simulink model "Plant_Simulation"  (R2024b)
settings: Solver=FixedStepAuto  StartTime=0.0  StopTime=10  FixedStep=5e-4  RelTol=1e-3
values from neighbouring files (symbols this model uses):
  ts = p.ctrl.ts_s    [discretization.m]
libraries: cstblocks x2
settings Model: Creator=HakvoortWBJ  LastModifiedBy=gicub
settings SolverCC: AlgebraicLoopSolver=TrustRegion
settings DataIOCC: ReturnWorkspaceOutputs=off
settings DebuggingCC: UnconnectedInputMsg=warning  UnconnectedOutputMsg=warning  UnconnectedLineMsg=warning  ArithmeticOperatorsInVariantConditions=warning
settings ModelReferenceCC: EnableRefExpFcnMdlSchedulingChecks=on
settings SFSimCC: CustomCodeUndefinedFunction=UseInterfaceOnly
settings RTWCC: GPUComputeCapability=3.5

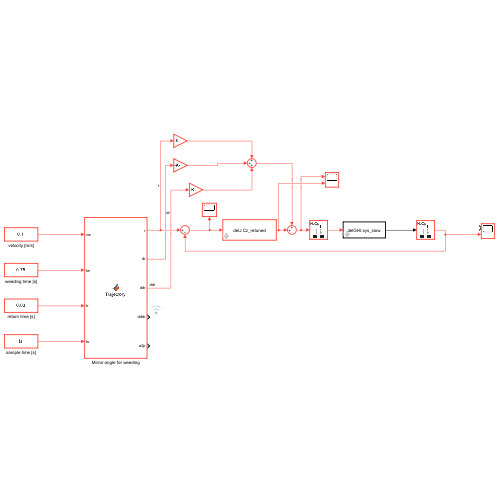
[thumbnail: Simulink's stored preview of the top-level diagram]
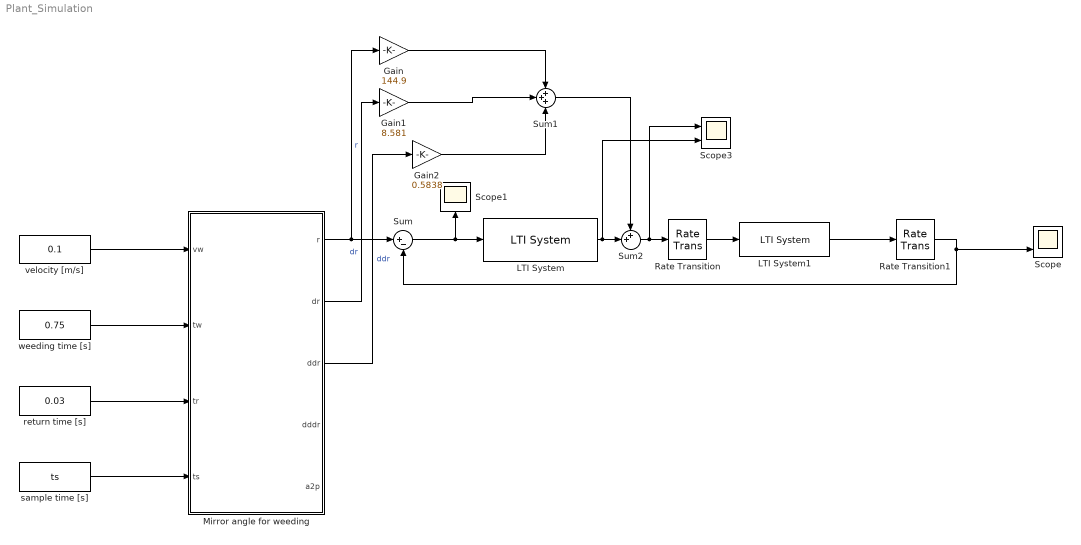
== system Plant_Simulation ==
  Gain : Gain  Gain=144.9
  Gain1 : Gain  Gain=8.581
  Gain2 : Gain  Gain=0.5838
  LTI System : cstblocks/LTI System  sys=delJ.Cz_retuned  IC=[]  PadeOrder=0
  LTI System1 : cstblocks/LTI System  sys=delGHI.sys_slow  IC=[]  PadeOrder=0
  Mirror angle for weeding : MATLAB Function  TreatAsAtomicUnit=on
  Rate Transition : RateTransition  OutPortSampleTimeOpt=Inherit
  Rate Transition1 : RateTransition  OutPortSampleTimeOpt=Inherit
  Scope : Scope  NumInputPorts=2
  Scope1 : Scope
  Scope3 : Scope  NumInputPorts=2
  Sum : Sum  Inputs=|+-
  Sum1 : Sum  Inputs=+++
  Sum2 : Sum  Inputs=++|
  return time [s] : Constant  Value=0.03  SampleTime=ts
  sample time [s] : Constant  Value=ts  SampleTime=ts
  velocity [m/s] : Constant  Value=0.1  SampleTime=ts
  weeding time [s] : Constant  Value=0.75  SampleTime=ts
  wires:
  velocity [m/s]/1 -> Mirror angle for weeding/1(vw)
  sample time [s]/1 -> Mirror angle for weeding/4(ts)
  return time [s]/1 -> Mirror angle for weeding/3(tr)
  weeding time [s]/1 -> Mirror angle for weeding/2(tw)
  Rate Transition/1 -> LTI System1/1
  Mirror angle for weeding/1(r) -> Gain/1, Sum/1  "r"
  Rate Transition1/1 -> Scope/2, Sum/2
  Sum/1 -> LTI System/1, Scope1/1
  Mirror angle for weeding/2(dr) -> Gain1/1  "dr"
  Mirror angle for weeding/3(ddr) -> Gain2/1  "ddr"
  Gain1/1 -> Sum1/2
  Gain/1 -> Sum1/1
  Gain2/1 -> Sum1/3
  Sum2/1 -> Scope3/1, Rate Transition/1
  LTI System/1 -> Scope3/2, Sum2/2
  Sum1/1 -> Sum2/1
  LTI System1/1 -> Rate Transition1/1

== matlab function Plant_Simulation/Mirror angle for weeding ==
  data: vw input; tw input; tr input; r output; dr output; ddr output; dddr output; ts input; a2p output
function [r, dr, ddr, dddr, a2p]   = Trajectory(vw, tw, tr, ts)
% Generates the mirror angle trajectory for weeding

% OUTPUTS:
% reference trajectory
% r:       [m]     position 
% dr:      [m/s]   velocity 
% ddr:     [m/s^2] acceleration
% dddr:    [m/s^3] jerk
% a2p:     [m]     angle to position transmission

% INPUTS
% vw:       [m/s]   driving velocity
% tw:       [s]     weeding time
% tr:       [s]     return time
% ts:       [s]     sample time

% define time 
persistent t
if isempty(t)
    t = 0;
end
% update time
t = mod(t+ts,tw+tr);  % [s] time
at = 2*pi/tr*t;       % [1/s] angle in period

% auxiliary variables
D = vw*(tw+tr);    % [m] maximum spot amplitude
xs = (D*tw)/(2*(tr + tw)) + (D*(1 - tw^2/(tr + tw)^2)^(1/2))/(2*pi) - (D*tw*acos(tw/(tr + tw)))/(2*pi*(tr + tw)); % [m] maximum amplitude
a2p = xs/17.5e-3;  % [m] angle to position transmission
Da = D/a2p;        % [rad] angular amplitude
va = vw/a2p;       % [rad/s] angular velocity

a = Da*tw/(tw+tr)/2; % [m] polynomial offset cofficient
b = -2*a/tr;         % [m/s] polynomial slope coefficient
c = Da/(2*pi);       % [m] sinusoidal amplitude

% compute angular trajectory and time derivatives
if t <= tr
    % sinusoidal return part
    r       = a+b*t+c*sin(at);
    dr      = b + c*2*pi/tr*cos(at);
    ddr     = -c*(2*pi/tr)^2*sin(at);
    dddr    = -c*(2*pi/tr)^3*cos(at);
else
    % constant velocity welding part
    r       = -Da*tw/(tw+tr)/2+(t-tr)*va;
    dr      = va;
    ddr     = 0;
    dddr    = 0;
end
